simulink model "GasTurbineSimulink"  (R2015b)
settings: Solver=VariableStepAuto  StartTime=0.0  StopTime=10.0  RelTol=1e-3
settings Model: Creator=GianAndrea  LastModifiedBy=GianAndrea

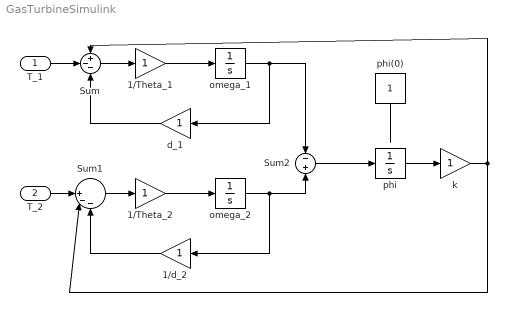
== system GasTurbineSimulink ==
  T_1 : Inport
  T_2 : Inport  Port=2
  1/Theta_1 : Gain
  1/Theta_2 : Gain
  1/d_2 : Gain
  Sum : Sum  Inputs=+--
  Sum1 : Sum  Inputs=||+--
  Sum2 : Sum  Inputs=-|+
  d_1 : Gain
  k : Gain
  omega_1 : Integrator
  omega_2 : Integrator
  phi : Integrator
  phi(0) : Constant
  wires:
  T_2/1 -> Sum1/1
  phi(0)/1 -> ?
  k/1 -> Sum/1, Sum1/2
  1/d_2/1 -> Sum1/3
  omega_1/1 -> d_1/1, Sum2/1
  omega_2/1 -> 1/d_2/1, Sum2/2
  1/Theta_2/1 -> omega_2/1
  Sum1/1 -> 1/Theta_2/1
  T_1/1 -> Sum/2
  Sum/1 -> 1/Theta_1/1
  1/Theta_1/1 -> omega_1/1
  d_1/1 -> Sum/3
  Sum2/1 -> phi/1
  phi/1 -> k/1
